simulink model "lorenz_sim"  (Simulink 8.1)
settings: Solver=ode45  StartTime=0.0  StopTime=10  RelTol=1e-3
values from neighbouring files (symbols this model uses):
  p = [10,8/3,28]    [Lorenz.m]
  x0 = [-8,8,27]    [Lorenz.m]
settings Model: Creator=trini  LastModifiedBy=trini
settings DataIOCC: SignalLoggingSaveFormat=Dataset
settings OptimizationCC: ExpressionDepthLimit=128
settings DebuggingCC: FcnCallInpInsideContextMsg=EnableAllAsError
settings GRTTargetCC: CombineOutputUpdateFcns=on  GRTInterface=off

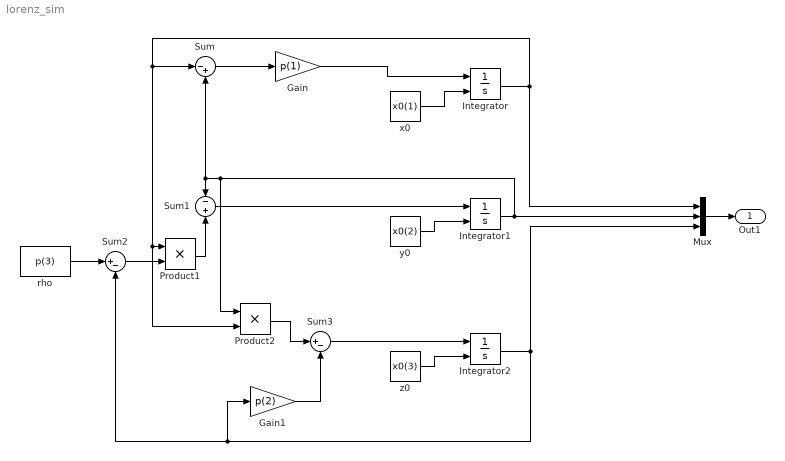
== system lorenz_sim ==
  Gain : Gain  Gain=p(1)
  Gain1 : Gain  Gain=p(2)
  Integrator : Integrator  InitialConditionSource=external
  Integrator1 : Integrator  InitialConditionSource=external
  Integrator2 : Integrator  InitialConditionSource=external
  Mux : Mux  Inputs=3
  Product1 : Product
  Product2 : Product
  Sum : Sum  Inputs=|-+
  Sum1 : Sum  Inputs=-+
  Sum2 : Sum  Inputs=|+-
  Sum3 : Sum  Inputs=|+-
  rho : Constant  Value=p(3)
  x0 : Constant  Value=x0(1)
  y0 : Constant  Value=x0(2)
  z0 : Constant  Value=x0(3)
  Out1 : Outport
  wires:
  x0/1 -> Integrator/2
  Gain/1 -> Integrator/1
  Sum/1 -> Gain/1
  Integrator/1 -> Sum/1, Product2/2, Product1/1, Mux/1
  y0/1 -> Integrator1/2
  Sum1/1 -> Integrator1/1
  Integrator1/1 -> Product2/1, Sum1/1, Sum/2, Mux/2
  rho/1 -> Sum2/1
  Product1/1 -> Sum1/2
  Sum2/1 -> Product1/2
  z0/1 -> Integrator2/2
  Integrator2/1 -> Gain1/1, Sum2/2, Mux/3
  Sum3/1 -> Integrator2/1
  Product2/1 -> Sum3/1
  Gain1/1 -> Sum3/2
  Mux/1 -> Out1/1
